simulink model "RemoteCHIL"  (Simulink 8.1)
settings: Solver=ode1  StartTime=0.0  StopTime=inf  FixedStep=Ts  MaxStep=1e-3  RelTol=1e-3
PostLoadFcn:
  | NREL_Mode=3; BANSHEE_init;
InitFcn:
  | NREL_Mode=3; BANSHEE_init;
values from neighbouring files (symbols this model uses):
  F4 = xlsread('F4_relay_nrel.xlsx')    [relay_settings_init.m]
  Ts = 100E-6    (= 0.0001)    [BANSHEE_init.m]    (also in Ghost_init.m)
undefined symbols (not defined in the file or in its folder): Left, Stim, type, V
libraries: simulink x50, relay_modbus_lib x11, simulink_extras x10, rtio_generic_modbus x6, rtlab x5, RMS_lib x4, cables_lib x3, relay_PLL_lib x3, PHIL_lib x2, breaker_lib x2, powerlib_extras x2, relay_ANSI_functions_lib x2
(part 1 of 3)
settings Model: ARTEMISmethode_block_infos=$$__separator__$$RemoteCHIL/ARTEMIS Guide$$__separator__$$  Creator=RE25624  LastModifiedBy=MGC4  BufferReuse=off
settings SolverCC: ZeroCrossAlgorithm=Adaptive
settings DataIOCC: ExternalInput=getinputstruct(op_snapshot1)  InitialState=getstatestruct(op_snapshot1)  LimitDataPoints=off  MaxDataPoints=90060  SignalLoggingSaveFormat=Dataset  SaveOutput=off  SignalLogging=off  DSMLogging=off  SaveTime=off  OutputSaveName=result
settings OptimizationCC: BlockReduction=off  OptimizeBlockIOStorage=off  BufferReuse=off  ExpressionFolding=off  LocalBlockOutputs=off
settings DebuggingCC: MaxConsecutiveZCsMsg=warning  IgnoredZcDiagnostic=none  SolverPrmCheckMsg=none  MultiTaskRateTransMsg=warning  ParameterPrecisionLossMsg=none  FcnCallInpInsideContextMsg=EnableAllAsWarning  FrameProcessingCompatibilityMsg=error  ModelReferenceExtraNoncontSigs=warning
settings ModelReferenceCC: UpdateModelReferenceTargets=IfOutOfDate
settings SFSimCC: SFSimEcho=off
settings GRTTargetCC: CodeReplacementLibrary=C89/C90 (ANSI)

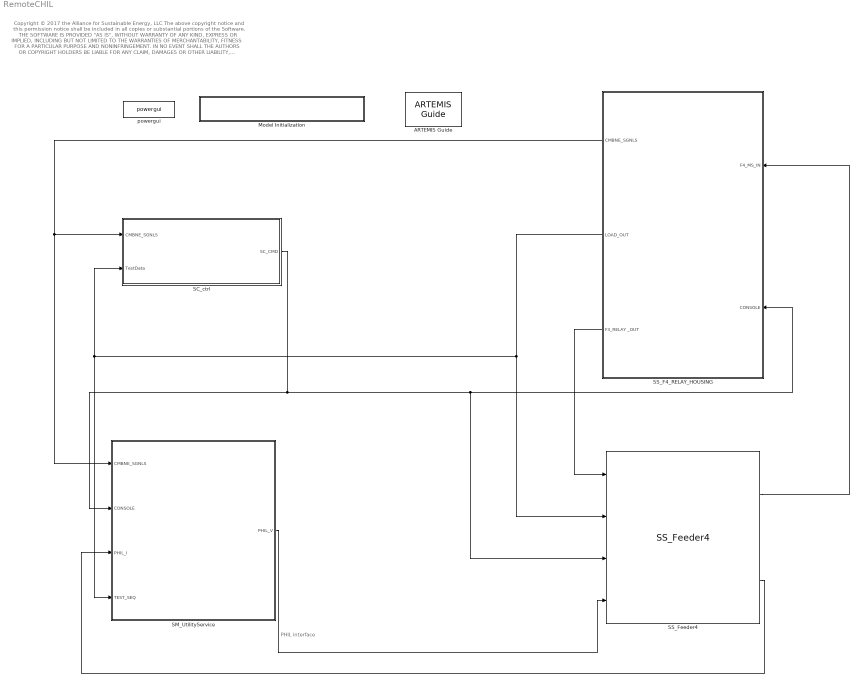
== system RemoteCHIL ==
  note: PHIL interface
  note: Copyright © 2017 the Alliance for Sustainable Energy, LLC
      |
      | The above copyright notice and this permission notice shall be included in all copies or substantial portions of the Software.
      |
      | THE SOFTWARE IS PROVIDED "AS IS", WITHOUT WARRANTY OF ANY KIND, EXPRESS OR IMPLIED, INCLUDING
      | BUT NOT LIMITED TO THE WARRANTIES OF MERCHANTABILITY, FITNESS FOR A PARTICULAR PURPOSE AND
      | NONINFRINGEMENT. IN NO EVENT SHALL THE AUTHORS OR COPYRIGHT HOLDERS BE LIABLE FOR ANY CLAIM,
      |  DAMAGES OR OTHER LIABILITY, WHETHER IN AN ACTION OF CONTRACT, TORT OR OTHERWISE, ARISING FROM,
      | OUT OF OR IN CONNECTION WITH THE SOFTWARE OR THE USE OR OTHER DEALINGS IN THE SOFTWARE
  ARTEMIS Guide : artemis/ARTEMIS/ARTEMIS Guide  Tag=FTSSmethode_opal_4hx0r99  Description=5.0_z1  lock=on  Ts=Ts  opt=art5  dyna=off  nb_perm=4  RT_fullcomp=off  ssn=on  ssn_itvc=off  ssn_ivic=off  ssn_ext=off  ssn_solver=Art5 with Backward Euler nodal interface  ssn_impulse=off  ssn_quasimpulse=off  ssn_impulse_loop=5  paraExtinctionThy=off  Thy_Impulse=on  dtc=Off  dtc_opt=normal  ao=on  simtype=off  ct_mac=off  lin_mov=off  lsp=[0.001 2]  spike_skip=Disabled  dtc_extra=1  dtc_sws=normal  dtc_pied=0.5  SPSRulesBlock=SPSRules  tre=on  ctmm=off  LF=off  dpl_type=ARTEMiS DPL  rlc_type=off  custom_type=off  para=on  ssn_ImpulseLoopBlockedStateUpdate=5  ssn_mov_iter_number=5  ssn_switch_iter_number=5  ssn_nib_type_verify=on
  Model Initialization : Subsystem  AncestorBlock=artemis/Tools /Misc/Model Initialization  mask(Model Functions){InitFcnX=NREL_Mode=3; BANSHEE_init;, prel=off, posl=on, inif=on, strf=off}
      mask prompts: InitFcnX "Initialisation"; prel "Preload Function"; posl "PostLoad Function"; inif "InitFcn"; strf "StartFcn"
      mask init:
      | currentBlock = gcb;
      | root = bdroot(currentBlock);
      | 
      | if ~strcmp(get_param(root,'BlockDiagramType'),'library')
      |     if prel==1
      |         set_param(root, 'PreLoadFcn', InitFcnX);
      |     else
      |         set_param(root, 'PreLoadFcn', '');
      |     end
      |     if inif==1
      |         set_param(root, 'InitFcn', InitFcnX);
      |     else
      |         set_param(root, 'InitFcn', '');
      |     end
      |     if strf==1
      |         set_param(root, 'StartFcn', InitFcnX);
      |     else
      |         set_param(root, 'StartFcn', '');
      |     end
      |     if posl==1
      |         set_param(root, 'PostLoadFcn', InitFcnX);
      |     else
      |         set_param(root, 'PostLoadFcn', '');
      |     end
      | end
      | 
      | pos = get_param(currentBlock, 'Position');
      | width = pos(3) - pos(1); height = pos(4) - pos(2);
      | txt = [ upper(root) '\n' '- InitFcn. . . . . '  get_param(root, 'InitFcn') ];
      settings: CopyFcn=set_param(gcb,'LinkStatus','inactive')
      mask Display: text(5, height*0.5, txt, 'horizontalAlignment', 'left', 'verticalAlignment', 'middle') ;
  SC_ctrl : Subsystem
  SM_UtilityService : Subsystem
  SS_F4_RELAY_HOUSING : Subsystem
  SS_Feeder4 : Feeder4_lib/SS_Feeder4
  powergui : powerlib/powergui  Priority=2  SimulationMode=Discrete  SolverType=Tustin  SampleTime=Ts  frequency=60  SPID=off  DisableSnubberDevices=off  DisableRonSwitches=off  DisableVfSwitches=off  SwTol=0  Interpol=off  DisplayEquations=off  frequencyindice=0  Pbase=100e6  ErrMax=1e-4  Iterations=50  UnitsV=kV  UnitsW=MW  FunctionMessages=off  echomessages=off  HookPort=off  EnableUseOfTLC=off  x0status=blocks  RestoreLinks=warning  ResistiveCurrentMeasurement=off  Frange=logspace(0,3,50)  Ylog=off  Xlog=off  ShowGrid=off  save=off  variable=ZData  structure=0  ZoomFFT=on  StartTime=0.0  cycles=2  DisplayStyle=off  fundamental=60  FreqAxis=off  MaxFrequency=1000  frequencyindicesteady=1  RmsSteady=1  display=off  Ts=0  methode=off
  wires:
  SS_Feeder4/1 -> SS_F4_RELAY_HOUSING/1(F4_MS_IN)
  SS_F4_RELAY_HOUSING/3(F3_RELAY _OUT) -> SS_Feeder4/1
  SS_F4_RELAY_HOUSING/2(LOAD_OUT) -> SC_ctrl/2(TestData), SM_UtilityService/4(TEST_SEQ), SS_Feeder4/2
  SS_F4_RELAY_HOUSING/1(CMBNE_SGNLS) -> SM_UtilityService/1(CMBNE_SGNLS), SC_ctrl/1(CMBNE_SGNLS)
  SC_ctrl/1(SC_CMD) -> SM_UtilityService/2(CONSOLE), SS_F4_RELAY_HOUSING/2(CONSOLE), SS_Feeder4/3
  SM_UtilityService/1(PHIL_V) -> SS_Feeder4/4
  SS_Feeder4/2 -> SM_UtilityService/3(PHIL_I)

== system RemoteCHIL/Model Initialization ==

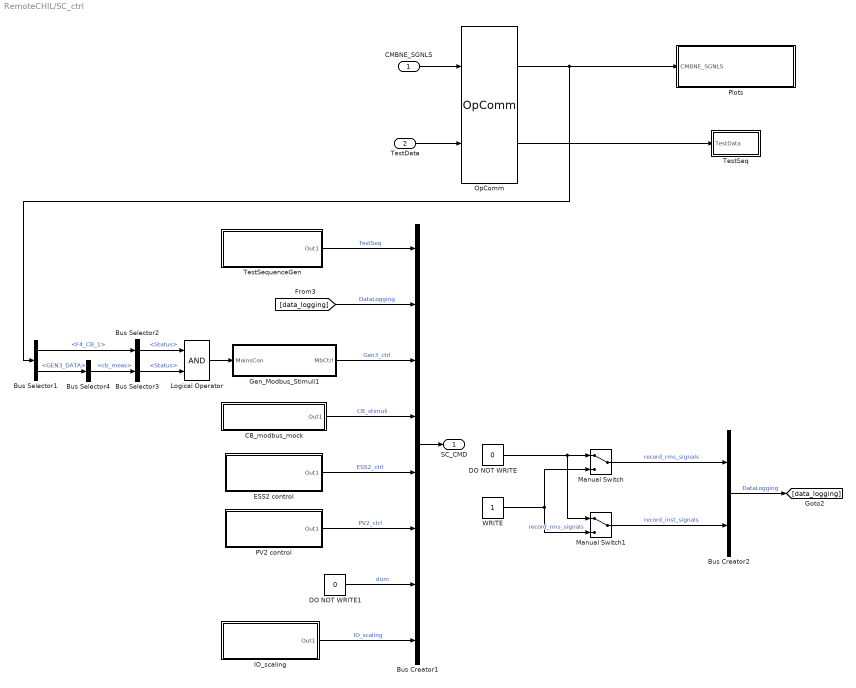
== system RemoteCHIL/SC_ctrl ==
  CMBNE_SGNLS : Inport
  TestData : Inport  Port=2
  Bus Creator1 : BusCreator  Inputs=8
  Bus Creator2 : BusCreator  Inputs=2
  Bus Selector1 : BusSelector  OutputSignals=F4_MS_IN.CB_DATA.F4_CB_1,F4_MS_IN.GEN3_DATA
  Bus Selector2 : BusSelector  OutputSignals=Status
  Bus Selector3 : BusSelector  OutputSignals=Status
  Bus Selector4 : BusSelector  OutputSignals=cb.cb_meas
  CB_modbus_mock : Subsystem
  DO NOT WRITE : Constant  Value=0
  DO NOT WRITE1 : Constant  Value=0
  ESS2 control : Subsystem
  Gen_Modbus_Stimuli1 : Subsystem
  IO_scaling : Subsystem
  Logical Operator : Logic  AllPortsSameDT=off  OutDataTypeStr=boolean
  Manual Switch : ManualSwitch
  Manual Switch1 : ManualSwitch
  OpComm : rtlab/OpComm  nbport=2  groupe_acq=1  subsys_rate=0  st=0  Synchronization=on  Interpolation=on  Threshold=1.0  Missed_Data=off  Sim_Time=off  Samples=off  dynSigOut=off  from_console=0  warning_done=off  writeOpCommFile=off  Offset=off
  PV2 control : Subsystem
  Plots : Subsystem
  TestSeq : Subsystem
  TestSequenceGen : Subsystem
  WRITE : Constant
  SC_CMD : Outport
  wires:
  CMBNE_SGNLS/1 -> OpComm/1
  Bus Creator1/1 -> SC_CMD/1
  Gen_Modbus_Stimuli1/1(MbCtrl) -> Bus Creator1/3  "Gen3_ctrl"
  Manual Switch/1 -> Bus Creator2/1  "record_rms_signals"
  Manual Switch1/1 -> Bus Creator2/2  "record_inst_signals"
  Bus Creator2/1 -> [data_logging]  "DataLogging"
  OpComm/2 -> TestSeq/1(TestData)
  TestData/1 -> OpComm/2
  WRITE/1 -> Manual Switch1/2, Manual Switch/2  "record_rms_signals"
  DO NOT WRITE/1 -> Manual Switch1/1, Manual Switch/1
  [data_logging] -> Bus Creator1/2  "DataLogging"
  CB_modbus_mock/1(Out1) -> Bus Creator1/4  "CB_stimuli"
  ESS2 control/1(Out1) -> Bus Creator1/5  "ESS2_ctrl"
  PV2 control/1(Out1) -> Bus Creator1/6  "PV2_ctrl"
  Logical Operator/1 -> Gen_Modbus_Stimuli1/1(MainsCon)
  OpComm/1 -> Bus Selector1/1, Plots/1(CMBNE_SGNLS)
  Bus Selector1/1 -> Bus Selector2/1  "<F4_CB_1>"
  Bus Selector1/2 -> Bus Selector4/1  "<GEN3_DATA>"
  Bus Selector2/1 -> Logical Operator/1  "<Status>"
  Bus Selector3/1 -> Logical Operator/2  "<Status>"
  Bus Selector4/1 -> Bus Selector3/1  "<cb_meas>"
  IO_scaling/1(Out1) -> Bus Creator1/8  "IO_scaling"
  TestSequenceGen/1(Out1) -> Bus Creator1/1  "TestSeq"
  DO NOT WRITE1/1 -> Bus Creator1/7  "dum"

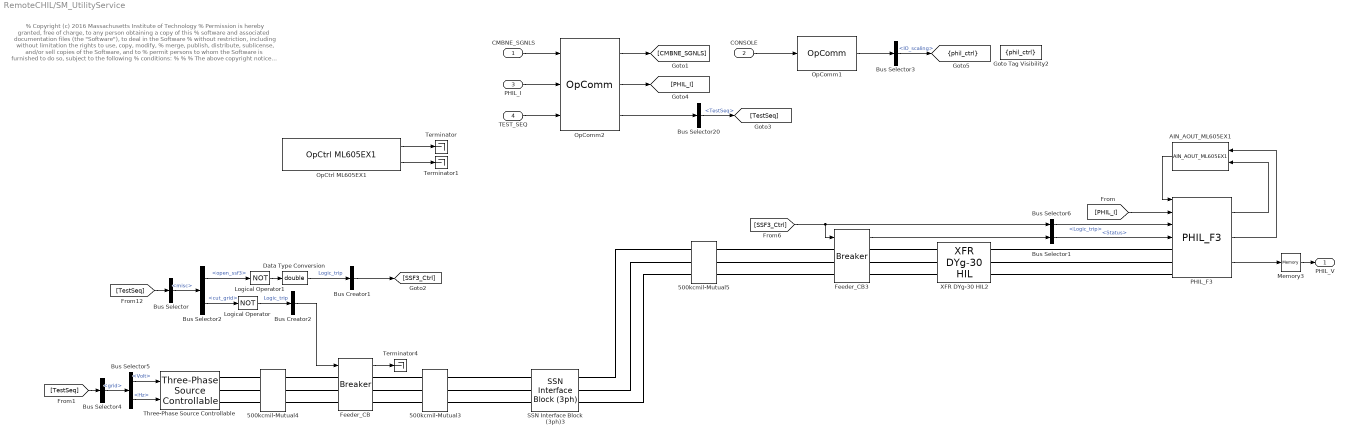
== system RemoteCHIL/SM_UtilityService ==
  note: % Copyright (c) 2016 Massachusetts Institute of Technology
      | % Permission is hereby granted, free of charge, to any person obtaining a copy of this
      | % software and associated documentation files (the "Software"), to deal in the Software
      | % without restriction, including without limitation the rights to use, copy, modify,
      | % merge, publish, distribute, sublicense, and/or sell copies of the Software, and to
      | % permit persons to whom the Software is furnished to do so, subject to the following
      | % conditions:
      | %
      | %
      | % The above copyright notice and this permission notice shall be included in
      | % all copies or substantial portions of the Software.
      | %
      | % THE SOFTWARE IS PROVIDED "AS IS", WITHOUT WARRANTY OF ANY KIND, EXPRESS OR IMPLIED,
      | % INCLUDING BUT NOT LIMITED TO THE WARRANTIES OF MERCHANTABILITY, FITNESS FOR A
      | % PARTICULAR PURPOSE AND NONINFRINGEMENT. IN NO EVENT SHALL THE AUTHORS OR COPYRIGHT
      | % HOLDERS BE LIABLE FOR ANY CLAIM, DAMAGES OR OTHER LIABILITY, WHETHER IN AN ACTION
      | % OF CONTRACT, TORT OR OTHERWISE, ARISING FROM, OUT OF OR IN CONNECTION WITH THE
      | % SOFTWARE OR THE USE OR OTHER DEALINGS IN THE SOFTWARE.
      | %
      | %
      | %%
  CMBNE_SGNLS : Inport
  CONSOLE : Inport  Port=2
  PHIL_I : Inport  Port=3
  TEST_SEQ : Inport  Port=4
  500kcmil-Mutual3 : cables_lib/500kcmil-Mutual  length=50  par_sets=1  ratio=3
  500kcmil-Mutual4 : cables_lib/500kcmil-Mutual  length=50  par_sets=1  ratio=3
  500kcmil-Mutual5 : cables_lib/500kcmil-Mutual  length=200  par_sets=1  ratio=3
  AIN_AOUT_ML605EX1 : PHIL_lib/AIN_AOUT_ML605EX1
  Bus Creator1 : BusCreator  Inputs=1
  Bus Creator2 : BusCreator  Inputs=1
  Bus Selector : BusSelector  OutputSignals=misc
  Bus Selector1 : BusSelector  OutputSignals=Status
  Bus Selector2 : BusSelector  OutputSignals=open_ssf3,cut_grid
  Bus Selector20 : BusSelector  OutputSignals=TestSeq
  Bus Selector3 : BusSelector  OutputSignals=IO_scaling
  Bus Selector4 : BusSelector  OutputSignals=grid
  Bus Selector5 : BusSelector  OutputSignals=Volt,Hz
  Bus Selector6 : BusSelector  OutputSignals=Logic_trip
  Data Type Conversion : DataTypeConversion  OutDataTypeStr=double
  Feeder_CB : breaker_lib/Breaker  Ts=Ts  mech_delay=cb_mech_delay
  Feeder_CB3 : breaker_lib/Breaker  Ts=Ts  mech_delay=cb_mech_delay
  Goto Tag Visibility2 : GotoTagVisibility  GotoTag=phil_ctrl
  Logical Operator : Logic  Operator=NOT  AllPortsSameDT=off  OutDataTypeStr=boolean
  Logical Operator1 : Logic  Operator=NOT  AllPortsSameDT=off  OutDataTypeStr=boolean
  Memory3 : Memory
  OpComm1 : rtlab/OpComm  nbport=1  groupe_acq=1  subsys_rate=0  st=0  Synchronization=on  Interpolation=on  Threshold=1.0  Missed_Data=off  Sim_Time=off  Samples=off  dynSigOut=off  from_console=1  warning_done=off  writeOpCommFile=off  Offset=off
  OpComm2 : rtlab/OpComm  nbport=3  groupe_acq=1  subsys_rate=0  st=0  Synchronization=on  Interpolation=on  Threshold=1.0  Missed_Data=off  Sim_Time=off  Samples=off  dynSigOut=off  from_console=0  warning_done=off  writeOpCommFile=off  Offset=off
  OpCtrl ML605EX1 : rtio_opalrt_ml605ex1/OpCtrl ML605EX1  CtrlName='ML605EX1 Ctrl'  boardid=4  BitstreamFilename=ML605_2-EX-0029-2_2_4_33-32AIO_16DIO16SelectableDIO-10-01.bin  numconfig=-1  mode=Master  externalClock=off  decimRtsi=0  calibIO=off  SampleTime=0  loadinport=-1
  PHIL_F3 : PHIL_lib/PHIL_F3
  SSN Interface Block (3ph)3 : ssn_lib/SSN Interface Block (3ph)  nb_phase=3  nb_port=2  p1_type=V-type(Left)  p2_type=V-type (Right)  p3_type=V-type(Left)  p4_type=V-type(Left)  p5_type=V-type(Left)  p6_type=V-type(Left)  p7_type=V-type(Left)  p8_type=V-type(Left)  p9_type=V-type(Left)  p10_type=V-type(Left)  p11_type=V-type(Left)  p12_type=V-type(Left)  p13_type=V-type(Left)  p14_type=V-type(Left)  p15_type=V-type(Left)  p16_type=V-type(Left)  I_port_shunt_resistance=1e9
  Terminator : Terminator
  Terminator1 : Terminator
  Terminator4 : Terminator
  Three-Phase Source Controllable : controllable_grid_lib/Three-Phase Source Controllable  Ts=Ts  Rg=0.8  Lg=16.58e-3
  XFR DYg-30 HIL2 : transformer_lib/XFR DYg-30 HIL  Rating=50000  Vp=115000  Vs=4160  Z=6  XR=30
  PHIL_V : Outport
  tag scope: phil_ctrl=scoped
  wires:
  CMBNE_SGNLS/1 -> OpComm2/1
  OpComm2/1 -> [CMBNE_SGNLS]
  CONSOLE/1 -> OpComm1/1
  OpComm1/1 -> Bus Selector3/1
  Feeder_CB/1 -> Terminator4/1
  Feeder_CB3/1 -> Bus Selector1/1
  Bus Selector20/1 -> [TestSeq]  "<TestSeq>"
  [TestSeq] -> Bus Selector/1
  Logical Operator/1 -> Bus Creator2/1  "Logic_trip"
  Bus Creator2/1 -> Feeder_CB/1
  PHIL_I/1 -> OpComm2/2
  OpComm2/2 -> [PHIL_I]
  TEST_SEQ/1 -> OpComm2/3
  OpComm2/3 -> Bus Selector20/1
  [SSF3_Ctrl] -> Bus Selector6/1, Feeder_CB3/1
  Memory3/1 -> PHIL_V/1
  Bus Selector1/1 -> PHIL_F3/4  "<Status>"
  PHIL_F3/3 -> Memory3/1
  Bus Selector6/1 -> PHIL_F3/3  "<Logic_trip>"
  [PHIL_I] -> PHIL_F3/2
  Bus Selector3/1 -> [phil_ctrl]  "<IO_scaling>"
  OpCtrl ML605EX1/1 -> Terminator/1
  OpCtrl ML605EX1/2 -> Terminator1/1
  Bus Selector/1 -> Bus Selector2/1  "<misc>"
  Bus Selector2/2 -> Logical Operator/1  "<cut_grid>"
  Bus Selector2/1 -> Logical Operator1/1  "<open_ssf3>"
  Logical Operator1/1 -> Data Type Conversion/1
  Bus Creator1/1 -> [SSF3_Ctrl]
  Data Type Conversion/1 -> Bus Creator1/1  "Logic_trip"
  [TestSeq] -> Bus Selector4/1
  Bus Selector4/1 -> Bus Selector5/1  "<grid>"
  Bus Selector5/2 -> Three-Phase Source Controllable/2  "<Hz>"
  Bus Selector5/1 -> Three-Phase Source Controllable/1  "<Volt>"
  AIN_AOUT_ML605EX1/1 -> PHIL_F3/1
  PHIL_F3/1 -> AIN_AOUT_ML605EX1/2
  PHIL_F3/2 -> AIN_AOUT_ML605EX1/1
  connections:
  500kcmil-Mutual3/LConn3 -- Feeder_CB/RConn3
  500kcmil-Mutual3/LConn1 -- Feeder_CB/RConn1
  500kcmil-Mutual3/LConn2 -- Feeder_CB/RConn2
  SSN Interface Block (3ph)3/LConn2 -- 500kcmil-Mutual3/RConn2
  SSN Interface Block (3ph)3/LConn1 -- 500kcmil-Mutual3/RConn1
  SSN Interface Block (3ph)3/LConn3 -- 500kcmil-Mutual3/RConn3
  500kcmil-Mutual4/RConn3 -- Feeder_CB/LConn3
  500kcmil-Mutual4/RConn2 -- Feeder_CB/LConn2
  500kcmil-Mutual4/RConn1 -- Feeder_CB/LConn1
  Three-Phase Source Controllable/RConn3 -- 500kcmil-Mutual4/LConn3
  Three-Phase Source Controllable/RConn1 -- 500kcmil-Mutual4/LConn1
  Three-Phase Source Controllable/RConn2 -- 500kcmil-Mutual4/LConn2
  500kcmil-Mutual5/LConn1 -- SSN Interface Block (3ph)3/RConn1
  500kcmil-Mutual5/LConn2 -- SSN Interface Block (3ph)3/RConn2
  500kcmil-Mutual5/LConn3 -- SSN Interface Block (3ph)3/RConn3
  Feeder_CB3/RConn2 -- XFR DYg-30 HIL2/LConn2
  Feeder_CB3/RConn1 -- XFR DYg-30 HIL2/LConn1
  Feeder_CB3/RConn3 -- XFR DYg-30 HIL2/LConn3
  500kcmil-Mutual5/RConn3 -- Feeder_CB3/LConn3
  500kcmil-Mutual5/RConn1 -- Feeder_CB3/LConn1
  500kcmil-Mutual5/RConn2 -- Feeder_CB3/LConn2
  PHIL_F3/LConn1 -- XFR DYg-30 HIL2/RConn1
  PHIL_F3/LConn2 -- XFR DYg-30 HIL2/RConn2
  PHIL_F3/LConn3 -- XFR DYg-30 HIL2/RConn3

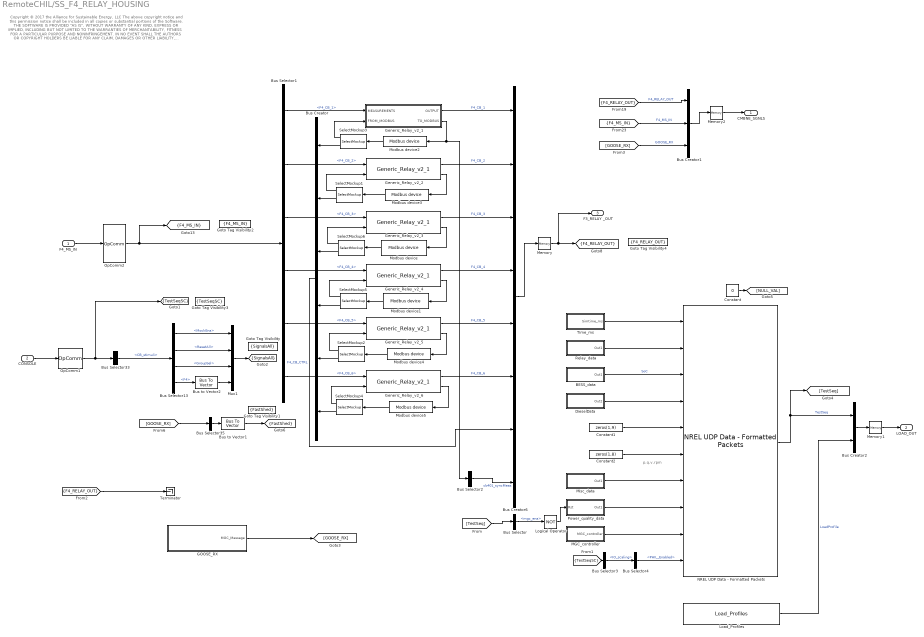
== system RemoteCHIL/SS_F4_RELAY_HOUSING ==
  note: p,q,v,rpm
  note: Copyright © 2017 the Alliance for Sustainable Energy, LLC
      |
      | The above copyright notice and this permission notice shall be included in all copies or substantial portions of the Software.
      |
      | THE SOFTWARE IS PROVIDED "AS IS", WITHOUT WARRANTY OF ANY KIND, EXPRESS OR IMPLIED, INCLUDING
      | BUT NOT LIMITED TO THE WARRANTIES OF MERCHANTABILITY, FITNESS FOR A PARTICULAR PURPOSE AND
      | NONINFRINGEMENT. IN NO EVENT SHALL THE AUTHORS OR COPYRIGHT HOLDERS BE LIABLE FOR ANY CLAIM,
      |  DAMAGES OR OTHER LIABILITY, WHETHER IN AN ACTION OF CONTRACT, TORT OR OTHERWISE, ARISING FROM,
      | OUT OF OR IN CONNECTION WITH THE SOFTWARE OR THE USE OR OTHER DEALINGS IN THE SOFTWARE
  F4_MS_IN : Inport
  CONSOLE : Inport  Port=2
  BESS_data : Subsystem
  Bus Creator : BusCreator  Inputs=6
  Bus Creator1 : BusCreator  Inputs=3
  Bus Creator2 : BusCreator  Inputs=2
  Bus Creator6 : BusCreator  Inputs=8
  Bus Selector : BusSelector  OutputSignals=misc.mgc_ena
  Bus Selector1 : BusSelector  OutputSignals=CB_DATA.F4_CB_1,CB_DATA.F4_CB_2,CB_DATA.F4_CB_3,CB_DATA.F4_CB_4,CB_DATA.F4_CB_5,CB_DATA.F4_CB_6
  Bus Selector13 : BusSelector  OutputSignals=MockEna,ResetAll,GroupSel,F4
  Bus Selector2 : BusSelector  OutputSignals=dF,dV,dWt  OutputAsBus=on
  Bus Selector3 : BusSelector  OutputSignals=IO_scaling
  Bus Selector33 : BusSelector  OutputSignals=CB_stimuli
  Bus Selector35 : BusSelector  OutputSignals=F4.CB401,F4.CB402,F4.CB403,NA,F4.CB405,F4.CB406  OutputAsBus=on
  Bus Selector4 : BusSelector  OutputSignals=PHIL_Enabled
  Bus to Vector1 : BusToVector
  Bus to Vector2 : BusToVector
  Constant : Constant  Value=0
  Constant1 : Constant  Value=zeros(1,9)
  Constant2 : Constant  Value=zeros(1,8)
  DieselData : Subsystem
  "GOOSE_RX " : Subsystem
  Generic_Relay_v2_1 : Subsystem  AncestorBlock=relay_modbus_lib/Generic_Relay_v2_1  mask(Generic Relay){Ts=Ts, relay_settings=[F4(1,:)]}
      mask prompts: Ts "Sampling Time [Sec]"; relay_settings "Relay Settings"
      mask help:
      | This relay simulates functions: synchronizing or synchronism-check (25), phase instantaneous overcurrent (50P), AC inverse time overcurrent (51P), undervoltage relay (27), and overvoltage relay (59).
      |
      | FEATURES:
      | 1) Receives commands from the microgrid controller via MODBUS/TCP
      | 2) Two groups of interchangeable protection settings
      |     - To be used for grid-tied and islanded protection modes
      | 3) Locked-out only enabled for functions (50P), (51P)
      |     - (27) and (59) pickups will be model inputs for the next revision
      | 4) MODBUS commands expected in the following order:
      |    a) Functions reset (Holding Reg# 2000)
      |    b) Breaker state   (Holding Reg# 2001)
      |    c) Protection mode (Holding Reg# 2002)
      |       - bit = 0; parameter group#1 (default)
      |       - bit = 1; parameter group#2
      |
      | See help or integration packet for further information.
      mask Help:
      | Procedure to reclose a breaker:
      | 1) reset all functions (Holding Reg# 2000)
      | 2) set breaker state (Holding Reg# 2001) to generate a close signal
      | 	- Synch-check (25) will automatically activate
      | 	- bit = 0, trip functions are active
      | 	- bit = 1, trip functions are not active
      | 
      | 
      | 
      | Field format/order for relay settings:
      | 	- Assuming zero delay between group settings changes
      | 
      | 1.  Relay#
      | 2.  Nominal VRMSLL
      | 3.  Max. Slip Voltage [%]
      | 4.  Max. Slip Angle [degree]
      | 5.  Max. Slip Frequency [Hz]
      | 6.  27P and 59P Trip Delay [Sec]
      | 7.  CT Primary
      | 
      | Parameter Group #1
      | 8.  50P Instantaneous overcurrent (IOC) Trip Pickup
      | 9.  50P IOC Trip Delay [sec]
      | 10.  51P Time overcurrent (TOC) Trip Pickup
      | 11.  51P Curve Type
      | 12.  51P TOC Time Dial
      | 13.  27P Trip Pickup [pu]
      | 14.  59P Trip Pickup [pu]
      | 
      | Parameter Group #2
      | 15.  50P IOC Trip Pickup
      | 16.  50P IOC Trip Delay [sec]
      | 17.  51P TOC Trip Pickup
      | 18.  51P Curve Type
      | 19.  51P TOC Time Dial
      | 20.  27P Trip Pickup [pu]
      | 21.  59P Trip Pickup [pu]
      | 
      | Available TCC Characteristics:
      | 	- The degree of inverseness for each curve approximates SEL-751
      | 
      | 51P Curve
      | 1: moderate inverse
      | 2: inverse
      | 3: very inverse
      | 4: extremely inverse
      | 
      | References:
      | [1] IEEE Std. C37.112-1996
      | [2] SEL 751 Instruction manual
      | [3] MIT-LL 2nd Microgrid Controller Symposium - Integration Packet
  Generic_Relay_v2_2 : relay_modbus_lib/Generic_Relay_v2_1  Ts=Ts  relay_settings=[F4(2,:)]
  Generic_Relay_v2_3 : relay_modbus_lib/Generic_Relay_v2_1  Ts=Ts  relay_settings=[F4(3,:)]
  Generic_Relay_v2_4 : relay_modbus_lib/Generic_Relay_v2_1  Ts=Ts  relay_settings=[F4(4,:)]
  Generic_Relay_v2_5 : relay_modbus_lib/Generic_Relay_v2_1  Ts=Ts  relay_settings=[F4(5,:)]
  Generic_Relay_v2_6 : relay_modbus_lib/Generic_Relay_v2_1  Ts=Ts  relay_settings=[F4(6,:)]
  Goto Tag Visibility : GotoTagVisibility  GotoTag=SignalsAll
  Goto Tag Visibility1 : GotoTagVisibility  GotoTag=FastShed
  Goto Tag Visibility2 : GotoTagVisibility  GotoTag=F4_MS_IN
  Goto Tag Visibility3 : GotoTagVisibility  GotoTag=TestSeqSC
  Goto Tag Visibility4 : GotoTagVisibility  GotoTag=F4_RELAY_OUT
  Load_Profiles : LoadProfiles_lib/Load_Profiles
  Logical Operator : Logic  Operator=NOT  AllPortsSameDT=off  OutDataTypeStr=boolean
  MGC_controller : Subsystem
  Memory : Memory
  Memory1 : Memory
  Memory2 : Memory
  Misc_data : Subsystem
  Modbus device : rtio_generic_modbus/Modbus device  conf_name=F4_relay_cfg3.opal  conf_name_mask=F4_relay_cfg3.xls  sample_time=Ts
  Modbus device1 : rtio_generic_modbus/Modbus device  conf_name=F4_relay_cfg4.opal  conf_name_mask=F4_relay_cfg4.xls  sample_time=Ts
  Modbus device2 : rtio_generic_modbus/Modbus device  conf_name=F4_relay_cfg1.opal  conf_name_mask=F4_relay_cfg1.xls  sample_time=Ts
  Modbus device3 : rtio_generic_modbus/Modbus device  conf_name=F4_relay_cfg2.opal  conf_name_mask=F4_relay_cfg2.xls  sample_time=Ts
  Modbus device4 : rtio_generic_modbus/Modbus device  conf_name=F4_relay_cfg5.opal  conf_name_mask=F4_relay_cfg5.xls  sample_time=Ts
  Modbus device5 : rtio_generic_modbus/Modbus device  conf_name=F4_relay_cfg6.opal  conf_name_mask=F4_relay_cfg6.xls  sample_time=Ts
  Mux1 : Mux
  NREL UDP Data - Formatted Packets : NREL_UDP_lib/NREL UDP Data - Formatted Packets  ProfileID=5  NumOfRelays=[59, [1, 1, 1000, 100]]  NumOfBatteries=2  NumOfDieselGensets=[2, [100, 100]]  NumOfNGCHPGensets=[1, [100, 100, 100, 100, 100, 100, 100, 100, 100]]  NumOfMotors=2  NumOfQuality=[23 10 10]  NumOfMiscellaneousDataScales=2  NumOfMiscellaneousDataSignalsScales=[[50, 1], [8, 1]]
  OpComm1 : rtlab/OpComm  nbport=1  groupe_acq=1  subsys_rate=0  st=0  Synchronization=on  Interpolation=on  Threshold=1.0  Missed_Data=off  Sim_Time=off  Samples=off  dynSigOut=off  from_console=1  warning_done=off  writeOpCommFile=off  Offset=off
  OpComm2 : rtlab/OpComm  nbport=1  groupe_acq=1  subsys_rate=0  st=0  Synchronization=on  Interpolation=on  Threshold=1.0  Missed_Data=off  Sim_Time=off  Samples=off  dynSigOut=off  from_console=0  warning_done=off  writeOpCommFile=off  Offset=off
  Power_quality_data : Subsystem
  Relay_data : Subsystem
  SelectMockup1 : relay_modbus_lib/SelectMockup  sigID=2  sigN=6
  SelectMockup2 : relay_modbus_lib/SelectMockup  sigID=5  sigN=6
  SelectMockup3 : relay_modbus_lib/SelectMockup  sigID=1  sigN=6
  SelectMockup4 : relay_modbus_lib/SelectMockup  sigID=6  sigN=6
  SelectMockup5 : relay_modbus_lib/SelectMockup  sigID=4  sigN=6
  SelectMockup6 : relay_modbus_lib/SelectMockup  sigID=3  sigN=6
  Terminator : Terminator
  Time_ms : Subsystem
  CMBNE_SGNLS : Outport
  LOAD_OUT : Outport  Port=2
  F3_RELAY _OUT : Outport  Port=3
  tag scope: F4_MS_IN=scoped, F4_RELAY_OUT=scoped, FastShed=scoped, SignalsAll=scoped, TestSeqSC=scoped
  wires:
  Load_Profiles/1 -> Bus Creator2/2  "LoadProfile"
  OpComm2/1 -> [F4_MS_IN], Bus Selector1/1
  Generic_Relay_v2_1/2(TO_MODBUS) -> Bus Selector2/1, Modbus device2/1
  F4_MS_IN/1 -> OpComm2/1
  Bus Selector1/1 -> Generic_Relay_v2_1/1(MEASUREMENTS)  "<F4_CB_1>"
  Bus Selector1/2 -> Generic_Relay_v2_2/1  "<F4_CB_2>"
  Bus Selector1/3 -> Generic_Relay_v2_3/1  "<F4_CB_3>"
  Bus Selector1/4 -> Generic_Relay_v2_4/1  "<F4_CB_4>"
  Bus Selector1/5 -> Generic_Relay_v2_5/1  "<F4_CB_5>"
  Bus Selector1/6 -> Generic_Relay_v2_6/1  "<F4_CB_6>"
  Generic_Relay_v2_1/1(OUTPUT) -> Bus Creator6/1  "F4_CB_1"
  Generic_Relay_v2_2/1 -> Bus Creator6/2  "F4_CB_2"
  Generic_Relay_v2_3/1 -> Bus Creator6/3  "F4_CB_3"
  Generic_Relay_v2_4/1 -> Bus Creator6/4  "F4_CB_4"
  Generic_Relay_v2_5/1 -> Bus Creator6/5  "F4_CB_5"
  Generic_Relay_v2_6/1 -> Bus Creator6/6  "F4_CB_6"
  Bus Creator6/1 -> Memory/1
  Memory/1 -> [F4_RELAY_OUT], F3_RELAY _OUT/1
  Memory1/1 -> LOAD_OUT/1
  Memory2/1 -> CMBNE_SGNLS/1
  Bus Creator1/1 -> Memory2/1
  [F4_RELAY_OUT] -> Bus Creator1/1  "F4_RELAY_OUT"
  [F4_MS_IN] -> Bus Creator1/2  "F4_MS_IN"
  CONSOLE/1 -> OpComm1/1
  OpComm1/1 -> [TestSeqSC], Bus Selector33/1
  Constant/1 -> [NULL_VAL]
  BESS_data/1(Out1) -> NREL UDP Data - Formatted Packets/3  "SoC"
  Constant2/1 -> NREL UDP Data - Formatted Packets/6
  Generic_Relay_v2_3/2 -> Modbus device/1
  Generic_Relay_v2_4/2 -> Modbus device1/1
  Modbus device2/1 -> SelectMockup3/1
  SelectMockup3/1 -> Generic_Relay_v2_1/2(FROM_MODBUS)
  Bus Selector33/1 -> Bus Selector13/1  "<CB_stimuli>"
  Bus Selector13/4 -> Bus to Vector2/1  "<F4>"
  Bus Selector13/1 -> Mux1/1  "<MockEna>"
  Bus to Vector2/1 -> Mux1/4
  Bus Selector13/3 -> Mux1/3  "<GroupSel>"
  Bus Selector13/2 -> Mux1/2  "<ResetAll>"
  Mux1/1 -> [SignalsAll]
  Generic_Relay_v2_2/2 -> Modbus device3/1
  Modbus device3/1 -> SelectMockup1/1
  SelectMockup1/1 -> Generic_Relay_v2_2/2
  Generic_Relay_v2_5/2 -> Modbus device4/1
  Modbus device4/1 -> SelectMockup2/1
  SelectMockup2/1 -> Generic_Relay_v2_5/2
  Generic_Relay_v2_6/2 -> Modbus device5/1
  Modbus device5/1 -> SelectMockup4/1
  SelectMockup4/1 -> Generic_Relay_v2_6/2
  Modbus device1/1 -> SelectMockup5/1
  SelectMockup5/1 -> Generic_Relay_v2_4/2
  SelectMockup6/1 -> Generic_Relay_v2_3/2
  Modbus device/1 -> SelectMockup6/1
  [GOOSE_RX] -> Bus Creator1/3  "GOOSE_RX"
  [GOOSE_RX] -> Bus Selector35/1
  Bus Selector35/1 -> Bus to Vector1/1
  Bus to Vector1/1 -> [FastShed]
  "GOOSE_RX "/1(MGC_Message) -> [GOOSE_RX]
  [F4_RELAY_OUT] -> Terminator/1
  Relay_data/1(Out1) -> NREL UDP Data - Formatted Packets/2
  Constant1/1 -> NREL UDP Data - Formatted Packets/5
  Misc_data/1(Out1) -> NREL UDP Data - Formatted Packets/7
  NREL UDP Data - Formatted Packets/1 -> [TestSeq], Bus Creator2/1  "TestSeq"
  Bus Creator2/1 -> Memory1/1
  Time_ms/1(Simtime_ms) -> NREL UDP Data - Formatted Packets/1
  DieselData/1(Out2) -> NREL UDP Data - Formatted Packets/4
  Power_quality_data/1(Out1) -> NREL UDP Data - Formatted Packets/8
  [TestSeq] -> Bus Selector/1
  Bus Selector/1 -> Logical Operator/1  "<mgc_ena>"
  Logical Operator/1 -> Power_quality_data/1(Rst)
  MGC_controller/1(MGC_controller) -> NREL UDP Data - Formatted Packets/9
  SelectMockup4/2 -> Bus Creator/6
  SelectMockup2/2 -> Bus Creator/5
  SelectMockup5/2 -> Bus Creator/4
  SelectMockup6/2 -> Bus Creator/3
  SelectMockup1/2 -> Bus Creator/2
  SelectMockup3/2 -> Bus Creator/1
  Bus Creator/1 -> Bus Creator6/7  "F4_CB_CTRL"
  Bus Selector2/1 -> Bus Creator6/8  "cb401_syncMeas"
  [TestSeqSC] -> Bus Selector3/1
  Bus Selector3/1 -> Bus Selector4/1  "<IO_scaling>"
  Bus Selector4/1 -> NREL UDP Data - Formatted Packets/10  "<PHIL_Enabled>"

== system RemoteCHIL/SC_ctrl/CB_modbus_mock ==
  note: Op_Mode:
      | 0 = Relay Functions
      | 1 = Close Breaker
      | 2 = Open Breaker
  note: Should be from pattern generator
  note: Copyright © 2017 the Alliance for Sustainable Energy, LLC
      |
      | The above copyright notice and this permission notice shall be included in all copies or substantial portions of the Software.
      |
      | THE SOFTWARE IS PROVIDED "AS IS", WITHOUT WARRANTY OF ANY KIND, EXPRESS OR IMPLIED, INCLUDING
      | BUT NOT LIMITED TO THE WARRANTIES OF MERCHANTABILITY, FITNESS FOR A PARTICULAR PURPOSE AND
      | NONINFRINGEMENT. IN NO EVENT SHALL THE AUTHORS OR COPYRIGHT HOLDERS BE LIABLE FOR ANY CLAIM,
      |  DAMAGES OR OTHER LIABILITY, WHETHER IN AN ACTION OF CONTRACT, TORT OR OTHERWISE, ARISING FROM,
      | OUT OF OR IN CONNECTION WITH THE SOFTWARE OR THE USE OR OTHER DEALINGS IN THE SOFTWARE
  Bus Creator1 : BusCreator
  Enabled : Constant
  F4 : Subsystem
  Manual Switch{,7..9} (4 alike) : ManualSwitch
  Manual Switch10 : ManualSwitch  CurrentSetting=0
  NO FAULT : Constant  Value=0
  NO FAULT2 : Constant  Value=0
  NO FAULT3 : Constant  Value=0
  Pulse Generator : DiscretePulseGenerator  SampleTime=[Stim.Ts Ts]
  RST : Constant
  Rate Transition : RateTransition  Deterministic=off
  setting #1 : Constant  Value=0
  setting #2 : Constant
  Out1 : Outport
  wires:
  Bus Creator1/1 -> Rate Transition/1
  F4/1(Out1) -> Bus Creator1/1  "F4"
  Manual Switch/1 -> Bus Creator1/2  "ResetAll"
  Manual Switch7/1 -> Manual Switch/2
  Pulse Generator/1 -> Manual Switch/1
  NO FAULT/1 -> Manual Switch7/1
  RST/1 -> Manual Switch7/2  "record_rms_signals"
  Manual Switch9/1 -> Manual Switch8/2
  NO FAULT2/1 -> Manual Switch8/1
  setting #1/1 -> Manual Switch9/1
  setting #2/1 -> Manual Switch9/2  "record_rms_signals"
  Manual Switch8/1 -> Bus Creator1/3  "GroupSel"
  Manual Switch10/1 -> Bus Creator1/4  "MockEna"
  NO FAULT3/1 -> Manual Switch10/1
  Enabled/1 -> Manual Switch10/2  "record_rms_signals"
  Rate Transition/1 -> Out1/1

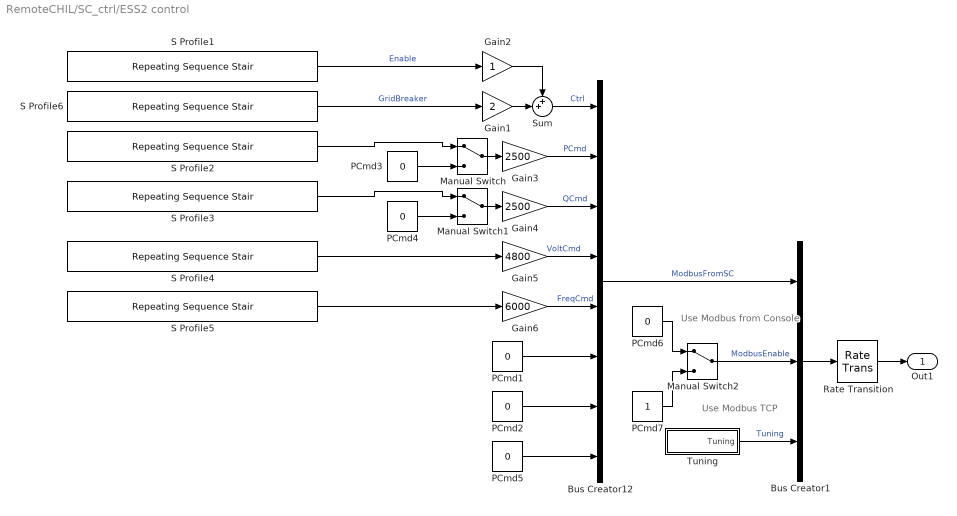
== system RemoteCHIL/SC_ctrl/ESS2 control ==
  note: Use Modbus from
      | Console
  note: Use Modbus TCP
  Bus Creator1 : BusCreator  Inputs=3
  Bus Creator12 : BusCreator  Inputs=8
  Gain1 : Gain  Gain=2
  Gain2 : Gain
  Gain3 : Gain  Gain=2500
  Gain4 : Gain  Gain=2500
  Gain5 : Gain  Gain=4800
  Gain6 : Gain  Gain=6000
  Manual Switch : ManualSwitch
  Manual Switch1 : ManualSwitch
  Manual Switch2 : ManualSwitch
  PCmd{1..6} (6 alike) : Constant  Value=0
  PCmd7 : Constant
  Rate Transition : RateTransition  Deterministic=off
  S Profile1 : simulink/Sources/Repeating Sequence Stair  OutValues=Stim.ESS2.Ena  tsamp=[Stim.Ts Ts]  OutMin=[]  OutMax=[]  OutDataTypeStr=Inherit: Inherit via back propagation  OutDataType=fixdt(0,8)  ConRadixGroup=Best Precision: Vector-wise  OutScaling=2^-12
  S Profile2 : simulink/Sources/Repeating Sequence Stair  OutValues=Stim.ESS2.p  tsamp=[Stim.Ts Ts]  OutMin=[]  OutMax=[]  OutDataTypeStr=Inherit: Inherit via back propagation  OutDataType=fixdt(0,8)  ConRadixGroup=Best Precision: Vector-wise  OutScaling=2^-12
  S Profile3 : simulink/Sources/Repeating Sequence Stair  OutValues=Stim.ESS2.q  tsamp=[Stim.Ts Ts]  OutMin=[]  OutMax=[]  OutDataTypeStr=Inherit: Inherit via back propagation  OutDataType=fixdt(0,8)  ConRadixGroup=Best Precision: Vector-wise  OutScaling=2^-12
  S Profile4 : simulink/Sources/Repeating Sequence Stair  OutValues=Stim.ESS2.v  tsamp=[Stim.Ts Ts]  OutMin=[]  OutMax=[]  OutDataTypeStr=Inherit: Inherit via back propagation  OutDataType=fixdt(0,8)  ConRadixGroup=Best Precision: Vector-wise  OutScaling=2^-12
  S Profile5 : simulink/Sources/Repeating Sequence Stair  OutValues=Stim.ESS2.f  tsamp=[Stim.Ts Ts]  OutMin=[]  OutMax=[]  OutDataTypeStr=Inherit: Inherit via back propagation  OutDataType=fixdt(0,8)  ConRadixGroup=Best Precision: Vector-wise  OutScaling=2^-12
  S Profile6 : simulink/Sources/Repeating Sequence Stair  OutValues=Stim.ESS2.VFmode  tsamp=[Stim.Ts Ts]  OutMin=[]  OutMax=[]  OutDataTypeStr=Inherit: Inherit via back propagation  OutDataType=fixdt(0,8)  ConRadixGroup=Best Precision: Vector-wise  OutScaling=2^-12
  Sum : Sum  Inputs=++|
  Tuning : Subsystem
  Out1 : Outport
  wires:
  S Profile6/1 -> Gain1/1  "GridBreaker"
  S Profile5/1 -> Gain6/1
  Manual Switch/1 -> Gain3/1
  Bus Creator12/1 -> Bus Creator1/1  "ModbusFromSC"
  Manual Switch1/1 -> Gain4/1
  S Profile1/1 -> Gain2/1  "Enable"
  S Profile4/1 -> Gain5/1
  PCmd4/1 -> Manual Switch1/2
  PCmd3/1 -> Manual Switch/2
  S Profile2/1 -> Manual Switch/1
  S Profile3/1 -> Manual Switch1/1
  Gain2/1 -> Sum/1
  Gain1/1 -> Sum/2
  Sum/1 -> Bus Creator12/1  "Ctrl"
  PCmd1/1 -> Bus Creator12/6
  PCmd2/1 -> Bus Creator12/7
  PCmd5/1 -> Bus Creator12/8
  Bus Creator1/1 -> Rate Transition/1
  Manual Switch2/1 -> Bus Creator1/2  "ModbusEnable"
  PCmd6/1 -> Manual Switch2/1
  PCmd7/1 -> Manual Switch2/2
  Gain3/1 -> Bus Creator12/2  "PCmd"
  Gain4/1 -> Bus Creator12/3  "QCmd"
  Gain5/1 -> Bus Creator12/4  "VoltCmd"
  Gain6/1 -> Bus Creator12/5  "FreqCmd"
  Rate Transition/1 -> Out1/1
  Tuning/1(Tuning) -> Bus Creator1/3  "Tuning"

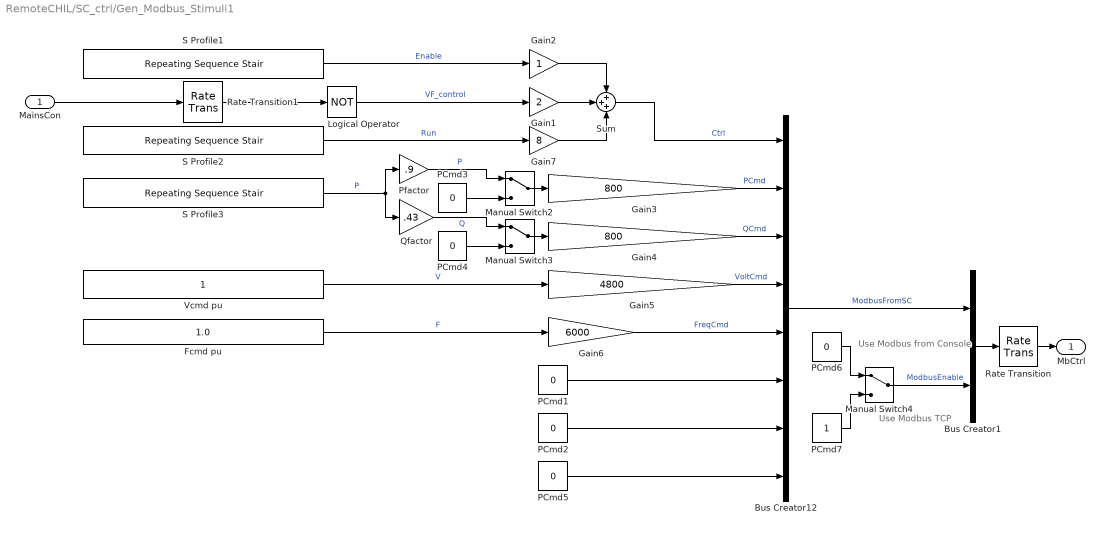
== system RemoteCHIL/SC_ctrl/Gen_Modbus_Stimuli1 ==
  note: Use Modbus from
      | Console
  note: Use Modbus TCP
  MainsCon : Inport
  Bus Creator1 : BusCreator  Inputs=2
  Bus Creator12 : BusCreator  Inputs=8
  Fcmd pu : Constant  Value=1.0
  Gain1 : Gain  Gain=2  OutDataTypeStr=double
  Gain2 : Gain
  Gain3 : Gain  Gain=800
  Gain4 : Gain  Gain=800
  Gain5 : Gain  Gain=4800
  Gain6 : Gain  Gain=6000
  Gain7 : Gain  Gain=8
  Logical Operator : Logic  Operator=NOT  AllPortsSameDT=off  OutDataTypeStr=boolean
  Manual Switch2 : ManualSwitch
  Manual Switch3 : ManualSwitch
  Manual Switch4 : ManualSwitch
  PCmd{1..6} (6 alike) : Constant  Value=0
  PCmd7 : Constant
  Pfactor : Gain  Gain=.9
  Qfactor : Gain  Gain=.43
  Rate Transition : RateTransition  Deterministic=off
  Rate Transition1 : RateTransition  Deterministic=off
  S Profile1 : simulink/Sources/Repeating Sequence Stair  OutValues=Stim.Gen3.Ena  tsamp=[Stim.Ts Ts]  OutMin=[]  OutMax=[]  OutDataTypeStr=Inherit: Inherit via back propagation  OutDataType=fixdt(0,8)  ConRadixGroup=Best Precision: Vector-wise  OutScaling=2^-12
  S Profile2 : simulink/Sources/Repeating Sequence Stair  OutValues=Stim.Gen3.Run  tsamp=[Stim.Ts Ts]  OutMin=[]  OutMax=[]  OutDataTypeStr=Inherit: Inherit via back propagation  OutDataType=fixdt(0,8)  ConRadixGroup=Best Precision: Vector-wise  OutScaling=2^-12
  S Profile3 : simulink/Sources/Repeating Sequence Stair  OutValues=Stim.Gen3.s  tsamp=[Stim.Ts Ts]  OutMin=[]  OutMax=[]  OutDataTypeStr=Inherit: Inherit via back propagation  OutDataType=fixdt(0,8)  ConRadixGroup=Best Precision: Vector-wise  OutScaling=2^-12
  Sum : Sum  Inputs=+++
  Vcmd pu : Constant
  MbCtrl : Outport
  wires:
  S Profile3/1 -> Pfactor/1, Qfactor/1  "P"
  Qfactor/1 -> Manual Switch3/1  "Q"
  Vcmd pu/1 -> Gain5/1  "V"
  Fcmd pu/1 -> Gain6/1  "F"
  Pfactor/1 -> Manual Switch2/1  "P"
  S Profile1/1 -> Gain2/1  "Enable"
  Manual Switch2/1 -> Gain3/1
  Bus Creator12/1 -> Bus Creator1/1  "ModbusFromSC"
  Manual Switch3/1 -> Gain4/1
  PCmd4/1 -> Manual Switch3/2
  PCmd3/1 -> Manual Switch2/2
  Gain2/1 -> Sum/1
  Gain1/1 -> Sum/2
  Sum/1 -> Bus Creator12/1  "Ctrl"
  PCmd1/1 -> Bus Creator12/6
  PCmd2/1 -> Bus Creator12/7
  PCmd5/1 -> Bus Creator12/8
  Bus Creator1/1 -> Rate Transition/1
  Manual Switch4/1 -> Bus Creator1/2  "ModbusEnable"
  PCmd6/1 -> Manual Switch4/1
  PCmd7/1 -> Manual Switch4/2
  Gain3/1 -> Bus Creator12/2  "PCmd"
  Gain4/1 -> Bus Creator12/3  "QCmd"
  Gain5/1 -> Bus Creator12/4  "VoltCmd"
  Gain6/1 -> Bus Creator12/5  "FreqCmd"
  S Profile2/1 -> Gain7/1  "Run"
  Gain7/1 -> Sum/3
  Logical Operator/1 -> Gain1/1  "VF_control"
  MainsCon/1 -> Rate Transition1/1
  Rate Transition/1 -> MbCtrl/1
  Rate Transition1/1 -> Logical Operator/1

== system RemoteCHIL/SC_ctrl/IO_scaling ==
  Bus Creator12 : BusCreator  Inputs=11
  Manual Switch : ManualSwitch
  PCmd1 : Constant  Value=1.015
  PCmd10 : Constant  Value=[1.1 0.8]
  PCmd2 : Constant  Value=125
  PCmd3 : Constant
  PCmd4 : Constant  Value=6
  PCmd5 : Constant  Value=[ 6 6 6 ]
  PCmd6 : Constant
  PCmd7 : Constant  Value=10/600
  PCmd8 : Constant  Value=0
  PCmd9 : Constant  Value=0
  Real_measurements : Constant
  Sim_measurements : Constant  Value=0
  Out1 : Outport
  wires:
  PCmd2/1 -> Bus Creator12/6  "I_sense_gain"
  Sim_measurements/1 -> Manual Switch/1
  Real_measurements/1 -> Manual Switch/2  "record_rms_signals"
  Manual Switch/1 -> Bus Creator12/5  "PHIL_Enabled"
  PCmd1/1 -> Bus Creator12/4  "AOUT_V_GAIN"
  PCmd3/1 -> Bus Creator12/1  "AIN_V_GAIN"
  PCmd6/1 -> Bus Creator12/2  "AIN_I_GAIN"
  Bus Creator12/1 -> Out1/1
  PCmd7/1 -> Bus Creator12/3  "AOUT_I_GAIN"
  PCmd4/1 -> Bus Creator12/7  "I_sense_offset"
  PCmd5/1 -> Bus Creator12/8  "I_gen_offset"
  PCmd9/1 -> Bus Creator12/9  "V_dq_mode_ena"
  PCmd10/1 -> Bus Creator12/10  "V_mag_limits"
  PCmd8/1 -> Bus Creator12/11  "Vang_enable"

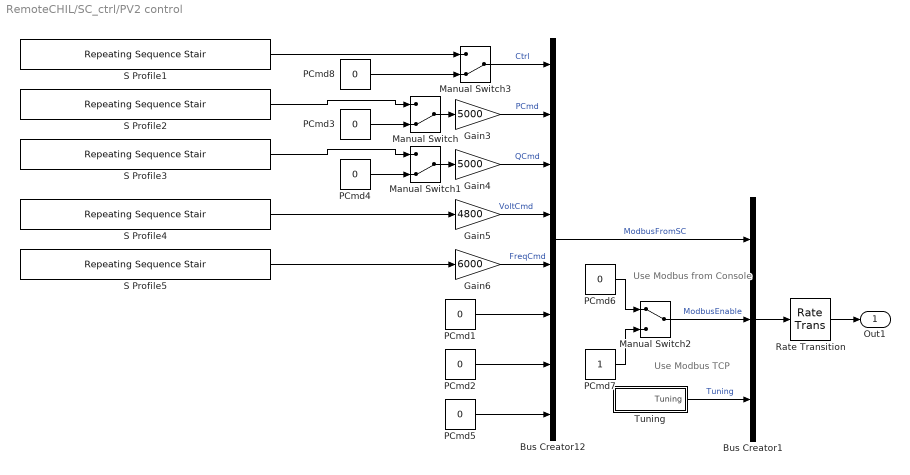
== system RemoteCHIL/SC_ctrl/PV2 control ==
  note: Use Modbus TCP
  note: Use Modbus from
      | Console
  Bus Creator1 : BusCreator  Inputs=3
  Bus Creator12 : BusCreator  Inputs=8
  Gain3 : Gain  Gain=5000
  Gain4 : Gain  Gain=5000
  Gain5 : Gain  Gain=4800
  Gain6 : Gain  Gain=6000
  Manual Switch : ManualSwitch  CurrentSetting=0
  Manual Switch1 : ManualSwitch  CurrentSetting=0
  Manual Switch2 : ManualSwitch
  Manual Switch3 : ManualSwitch  CurrentSetting=0
  PCmd{1..6,8} (7 alike) : Constant  Value=0
  PCmd7 : Constant
  Rate Transition : RateTransition  Deterministic=off
  S Profile1 : simulink/Sources/Repeating Sequence Stair  OutValues=Stim.PV2.Ena  tsamp=[Stim.Ts Ts]  OutMin=[]  OutMax=[]  OutDataTypeStr=Inherit: Inherit via back propagation  OutDataType=fixdt(0,8)  ConRadixGroup=Best Precision: Vector-wise  OutScaling=2^-12
  S Profile2 : simulink/Sources/Repeating Sequence Stair  OutValues=Stim.ESS2.p  tsamp=[Stim.Ts Ts]  OutMin=[]  OutMax=[]  OutDataTypeStr=Inherit: Inherit via back propagation  OutDataType=fixdt(0,8)  ConRadixGroup=Best Precision: Vector-wise  OutScaling=2^-12
  S Profile3 : simulink/Sources/Repeating Sequence Stair  OutValues=Stim.ESS2.q  tsamp=[Stim.Ts Ts]  OutMin=[]  OutMax=[]  OutDataTypeStr=Inherit: Inherit via back propagation  OutDataType=fixdt(0,8)  ConRadixGroup=Best Precision: Vector-wise  OutScaling=2^-12
  S Profile4 : simulink/Sources/Repeating Sequence Stair  OutValues=Stim.ESS2.v  tsamp=[Stim.Ts Ts]  OutMin=[]  OutMax=[]  OutDataTypeStr=Inherit: Inherit via back propagation  OutDataType=fixdt(0,8)  ConRadixGroup=Best Precision: Vector-wise  OutScaling=2^-12
  S Profile5 : simulink/Sources/Repeating Sequence Stair  OutValues=Stim.ESS2.f  tsamp=[Stim.Ts Ts]  OutMin=[]  OutMax=[]  OutDataTypeStr=Inherit: Inherit via back propagation  OutDataType=fixdt(0,8)  ConRadixGroup=Best Precision: Vector-wise  OutScaling=2^-12
  Tuning : Subsystem
  Out1 : Outport
  wires:
  Rate Transition/1 -> Out1/1
  Gain6/1 -> Bus Creator12/5  "FreqCmd"
  Gain5/1 -> Bus Creator12/4  "VoltCmd"
  Gain4/1 -> Bus Creator12/3  "QCmd"
  Gain3/1 -> Bus Creator12/2  "PCmd"
  PCmd7/1 -> Manual Switch2/2
  PCmd6/1 -> Manual Switch2/1
  Manual Switch2/1 -> Bus Creator1/2  "ModbusEnable"
  Bus Creator1/1 -> Rate Transition/1
  PCmd5/1 -> Bus Creator12/8
  PCmd2/1 -> Bus Creator12/7
  PCmd1/1 -> Bus Creator12/6
  S Profile1/1 -> Manual Switch3/1
  S Profile3/1 -> Manual Switch1/1
  S Profile2/1 -> Manual Switch/1
  PCmd3/1 -> Manual Switch/2
  PCmd4/1 -> Manual Switch1/2
  S Profile4/1 -> Gain5/1
  Manual Switch1/1 -> Gain4/1
  Bus Creator12/1 -> Bus Creator1/1  "ModbusFromSC"
  Manual Switch/1 -> Gain3/1
  S Profile5/1 -> Gain6/1
  PCmd8/1 -> Manual Switch3/2
  Manual Switch3/1 -> Bus Creator12/1  "Ctrl"
  Tuning/1(Tuning) -> Bus Creator1/3  "Tuning"

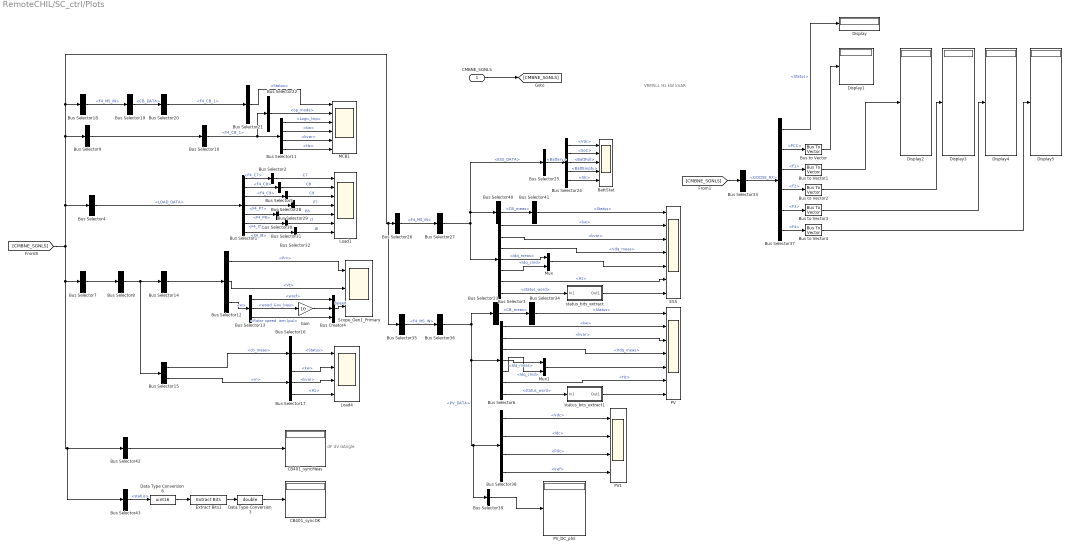
== system RemoteCHIL/SC_ctrl/Plots ==
  note: dF
      | dV
      | dAngle
  note: VRMSLL
      |  Hz
      | kW
      | kVAR
  CMBNE_SGNLS : Inport
  BattStat : Scope  NumInputPorts=5
      settings: YMin=-1~-1~-1~49.9984~-5  YMax=1~1~1~49.9985~5  SaveName=ScopeData11  Decimation=Stim.Dec
  Bus Creator4 : BusCreator  Inputs=3
  Bus Selector1 : BusSelector  OutputSignals=F4_C7,F4_C8,F4_C9,F4_P7,F4_P8,F4_I7,F4_I8
  Bus Selector10 : BusSelector  OutputSignals=F4_CB_1
  Bus Selector11 : BusSelector  OutputSignals=Logic_trip,m.kw,m.kvar,m.Hz
  Bus Selector12 : BusSelector  OutputSignals=Pm,Vt,w
  Bus Selector13 : BusSelector  OutputSignals="wref,w.wood_Gov_bias,w.Rotor speed  wm (pu)"
  Bus Selector14 : BusSelector  OutputSignals=gen  OutputAsBus=on
  Bus Selector15 : BusSelector  OutputSignals=cb.cb_meas,cb.relay_out.m
  Bus Selector16 : BusSelector  OutputSignals=Status
  Bus Selector17 : BusSelector  OutputSignals=kw,kvar,Hz
  Bus Selector18 : BusSelector  OutputSignals=F4_MS_IN
  Bus Selector19 : BusSelector  OutputSignals=CB_DATA
  Bus Selector{2,5,28..32} (7 alike) : BusSelector  OutputSignals=kw  OutputAsBus=on
  Bus Selector20 : BusSelector  OutputSignals=F4_CB_1
  Bus Selector21 : BusSelector  OutputSignals=Status
  Bus Selector22 : BusSelector  OutputSignals=op_mode
  Bus Selector23 : BusSelector  OutputSignals=CB_meas
  Bus Selector24 : BusSelector  OutputSignals=Vdc,SoC,BattFull,BattEmpty,Idc
  Bus Selector25 : BusSelector  OutputSignals=Battery
  Bus Selector26 : BusSelector  OutputSignals=F4_MS_IN
  Bus Selector27 : BusSelector  OutputSignals=ESS_DATA
  Bus Selector3 : BusSelector  OutputSignals=CB_meas.relay_out.m.kw,CB_meas.relay_out.m.kvar,Inverter.Vdq_meas,Inverter.Idq_meas,Inverter.Idq_cmd,CB_meas.relay_out.m.Hz,status_word
  Bus Selector33 : BusSelector  OutputSignals=GOOSE_RX
  Bus Selector34 : BusSelector  OutputSignals=cb_meas.Status
  Bus Selector35 : BusSelector  OutputSignals=F4_MS_IN
  Bus Selector36 : BusSelector  OutputSignals=PV_DATA
  Bus Selector37 : BusSelector  OutputSignals=Status,PCC,F1,F2,F3,F4
  Bus Selector38 : BusSelector  OutputSignals=pv_phil.Vdc,pv_phil.Idc,pv_phil.Pdc,pv_phil.Iref
  Bus Selector39 : BusSelector  OutputSignals=pv_phil.Vdc,pv_phil.Idc,pv_phil.Pdc,pv_phil.Iref  OutputAsBus=on
  Bus Selector4 : BusSelector  OutputSignals=F4_MS_IN.LOAD_DATA
  Bus Selector40 : BusSelector  OutputSignals=CB_meas
  Bus Selector41 : BusSelector  OutputSignals=cb_meas.Status
  Bus Selector42 : BusSelector  OutputSignals=F4_RELAY_OUT.cb401_syncMeas.dF,F4_RELAY_OUT.cb401_syncMeas.dV,F4_RELAY_OUT.cb401_syncMeas.dWt  OutputAsBus=on
  Bus Selector43 : BusSelector  OutputSignals=F4_RELAY_OUT.F4_CB_1.m.status
  Bus Selector6 : BusSelector  OutputSignals=CB_meas.relay_out.m.kw,CB_meas.relay_out.m.kvar,Inverter.Vdq_meas,Inverter.Idq_meas,Inverter.Idq_cmd,CB_meas.relay_out.m.Hz,status_word
  Bus Selector7 : BusSelector  OutputSignals=F4_MS_IN  OutputAsBus=on
  Bus Selector8 : BusSelector  OutputSignals=GEN3_DATA  OutputAsBus=on
  Bus Selector9 : BusSelector  OutputSignals=F4_RELAY_OUT  OutputAsBus=on
  Bus to Vector{,1..4} (5 alike) : BusToVector
  CB401_syncMeas : Display
  CB401_syncOK : Display
  Data Type Conversion3 : DataTypeConversion  OutDataTypeStr=double
  Data Type Conversion6 : DataTypeConversion  OutDataTypeStr=uint16
  Display{,1..5} (6 alike) : Display
  ESS : Scope  NumInputPorts=7
      settings: YMin=-1~-1.81789e-64~-4.43008e-63~-2.5e-15~-3e-30~57~-5  YMax=1~-1.64475e-64~-4.00816e-63~3e-15~2.5e-30~63~5  SaveName=ScopeData13  Decimation=Stim.Dec
  Extract Bits1 : simulink/Logic and Bit Operations/Extract Bits  bitsToExtract=Range of bits  numBits=8  bitIdxRange=1  outScalingMode=Treat bit field as an integer
  Gain : Gain  Gain=10
  Load1 : Scope  NumInputPorts=7
      settings: YMin=0~-5~-400~0~-0.25~58.5~-5  YMax=1~5~400~2.75~1.25~62.5~5  SaveName=ScopeData2  Decimation=Stim.Dec
  Load4 : Scope  NumInputPorts=4
      settings: YMin=0.95~-150~-500~-500  YMax=1.05~150~500~500  SaveName=ScopeData6  Decimation=Stim.Dec
  MCB1 : Scope  NumInputPorts=6
      settings: YMin=-1~2~-1~-5.20939e+238~-1.2e+239~60.125  YMax=1~2~1~9e+254~1e+238~60.3  SaveName=ScopeData7  Decimation=Stim.Dec
  Mux : Mux  Inputs=2
  Mux1 : Mux  Inputs=2
  PV : Scope  NumInputPorts=7
      settings: YMin=-1~-6.51427e-30~-1.68788e-28~0~-4e-13~57~-5  YMax=1~-5.89387e-30~-1.52712e-28~400~5e-14~63~5  SaveName=ScopeData3  Decimation=Stim.Dec
  PV1 : Scope  NumInputPorts=4
      settings: YMin=-1~-6.51427e-30~-1.68788e-28~0  YMax=1~-5.89387e-30~-1.52712e-28~400  Decimation=Stim.Dec
  PV_DC_phil : Display
  Scope_Gen1_Primary : Scope  NumInputPorts=3
      settings: ShowLegends=on  YMin=0.55~2.77556e-17~-0.9  YMax=1.35~1.1~1.1  SaveName=ScopeData5  Decimation=Stim.Dec
  status_bits_extract : Subsystem
  status_bits_extract1 : Subsystem
  wires:
  CMBNE_SGNLS/1 -> [CMBNE_SGNLS]
  Bus Selector9/1 -> Bus Selector10/1
  Bus Selector7/1 -> Bus Selector8/1
  Bus Selector8/1 -> Bus Selector15/1, Bus Selector14/1
  Bus Selector12/1 -> Scope_Gen1_Primary/1  "<Pm>"
  Bus Selector12/2 -> Scope_Gen1_Primary/2  "<Vt>"
  Bus Selector12/3 -> Bus Selector13/1  "<w>"
  Bus Selector13/1 -> Bus Creator4/1  "<wref>"
  Bus Selector13/2 -> Gain/1  "<wood_Gov_bias>"
  Bus Selector13/3 -> Bus Creator4/3  "<Rotor speed  wm (pu)>"
  Gain/1 -> Bus Creator4/2
  Bus Creator4/1 -> Scope_Gen1_Primary/3  "Speed"
  Bus Selector14/1 -> Bus Selector12/1
  Bus Selector15/1 -> Bus Selector16/1  "<cb_meas>"
  Bus Selector16/1 -> Load4/1  "<Status>"
  Bus Selector15/2 -> Bus Selector17/1  "<m>"
  Bus Selector17/1 -> Load4/2  "<kw>"
  Bus Selector17/2 -> Load4/3  "<kvar>"
  Bus Selector17/3 -> Load4/4  "<Hz>"
  Bus Selector18/1 -> Bus Selector19/1  "<F4_MS_IN>"
  Bus Selector19/1 -> Bus Selector20/1  "<CB_DATA>"
  Bus Selector20/1 -> Bus Selector21/1  "<F4_CB_1>"
  Bus Selector21/1 -> MCB1/1  "<Status>"
  Bus Selector10/1 -> Bus Selector22/1, Bus Selector11/1  "<F4_CB_1>"
  Bus Selector22/1 -> MCB1/2  "<op_mode>"
  Bus Selector3/4 -> Mux/1  "<Idq_meas>"
  Mux/1 -> ESS/5
  Bus Selector3/3 -> ESS/4  "<Vdq_meas>"
  Bus Selector24/2 -> BattStat/2  "<SoC>"
  Bus Selector24/1 -> BattStat/1  "<Vdc>"
  Bus Selector24/3 -> BattStat/3  "<BattFull>"
  Bus Selector24/4 -> BattStat/4  "<BattEmpty>"
  Bus Selector25/1 -> Bus Selector24/1  "<Battery>"
  Bus Selector3/5 -> Mux/2  "<Idq_cmd>"
  Bus Selector3/6 -> ESS/6  "<Hz>"
  Bus Selector26/1 -> Bus Selector27/1  "<F4_MS_IN>"
  Bus Selector11/1 -> MCB1/3  "<Logic_trip>"
  Bus Selector11/2 -> MCB1/4  "<kw>"
  Bus Selector11/3 -> MCB1/5  "<kvar>"
  Bus Selector11/4 -> MCB1/6  "<Hz>"
  Bus Selector1/1 -> Bus Selector2/1  "<F4_C7>"
  Bus Selector2/1 -> Load1/1  "C7"
  Bus Selector1/2 -> Bus Selector5/1  "<F4_C8>"
  Bus Selector5/1 -> Load1/2  "C8"
  Bus Selector1/3 -> Bus Selector28/1  "<F4_C9>"
  Bus Selector28/1 -> Load1/3  "C9"
  Bus Selector1/4 -> Bus Selector29/1  "<F4_P7>"
  Bus Selector29/1 -> Load1/4  "P7"
  Bus Selector30/1 -> Load1/5  "P8"
  Bus Selector31/1 -> Load1/6  "I7"
  Bus Selector1/7 -> Bus Selector32/1  "<F4_I8>"
  Bus Selector32/1 -> Load1/7  "I8"
  Bus Selector3/1 -> ESS/2  "<kw>"
  Bus Selector3/2 -> ESS/3  "<kvar>"
  [CMBNE_SGNLS] -> Bus Selector4/1, Bus Selector35/1, Bus Selector26/1, Bus Selector18/1, Bus Selector9/1, Bus Selector43/1, Bus Selector42/1, Bus Selector7/1
  Bus Selector6/4 -> Mux1/1  "<Idq_meas>"
  Mux1/1 -> PV/5
  Bus Selector6/3 -> PV/4  "<Vdq_meas>"
  Bus Selector6/5 -> Mux1/2  "<Idq_cmd>"
  Bus Selector6/6 -> PV/6  "<Hz>"
  Bus Selector35/1 -> Bus Selector36/1  "<F4_MS_IN>"
  Bus Selector6/1 -> PV/2  "<kw>"
  Bus Selector6/2 -> PV/3  "<kvar>"
  Bus Selector1/5 -> Bus Selector30/1  "<F4_P8>"
  Bus Selector1/6 -> Bus Selector31/1  "<F4_I7>"
  Bus Selector36/1 -> Bus Selector23/1, Bus Selector39/1, Bus Selector38/1, Bus Selector6/1  "<PV_DATA>"
  Bus Selector34/1 -> PV/1  "<Status>"
  Bus Selector23/1 -> Bus Selector34/1  "<CB_meas>"
  Bus Selector27/1 -> Bus Selector25/1, Bus Selector40/1, Bus Selector3/1  "<ESS_DATA>"
  Bus Selector41/1 -> ESS/1  "<Status>"
  Bus Selector40/1 -> Bus Selector41/1  "<CB_meas>"
  Bus Selector24/5 -> BattStat/5  "<Idc>"
  status_bits_extract/1(Out1) -> ESS/7
  Bus Selector6/7 -> status_bits_extract1/1(In1)  "<status_word>"
  status_bits_extract1/1(Out1) -> PV/7
  Bus Selector3/7 -> status_bits_extract/1(In1)  "<status_word>"
  Bus Selector4/1 -> Bus Selector1/1  "<LOAD_DATA>"
  [CMBNE_SGNLS] -> Bus Selector33/1
  Bus Selector33/1 -> Bus Selector37/1  "<GOOSE_RX>"
  Bus Selector37/1 -> Display/1  "<Status>"
  Bus Selector37/2 -> Bus to Vector/1  "<PCC>"
  Bus to Vector/1 -> Display1/1
  Bus Selector37/3 -> Bus to Vector1/1  "<F1>"
  Bus Selector37/6 -> Bus to Vector4/1  "<F4>"
  Bus Selector37/5 -> Bus to Vector3/1  "<F3>"
  Bus Selector37/4 -> Bus to Vector2/1  "<F2>"
  Bus to Vector4/1 -> Display5/1
  Bus to Vector3/1 -> Display4/1
  Bus to Vector2/1 -> Display3/1
  Bus to Vector1/1 -> Display2/1
  Bus Selector38/1 -> PV1/1  "<Vdc>"
  Bus Selector38/2 -> PV1/2  "<Idc>"
  Bus Selector38/3 -> PV1/3  "<Pdc>"
  Bus Selector38/4 -> PV1/4  "<Iref>"
  Bus Selector39/1 -> PV_DC_phil/1
  Bus Selector42/1 -> CB401_syncMeas/1
  Bus Selector43/1 -> Data Type Conversion6/1  "<status>"
  Extract Bits1/1 -> Data Type Conversion3/1
  Data Type Conversion6/1 -> Extract Bits1/1
  Data Type Conversion3/1 -> CB401_syncOK/1
